simulink model "risingEdge"  (R2024a)
settings: Solver=FixedStepDiscrete  StartTime=0.0  StopTime=10.0  RelTol=1e-3
undefined symbols (not defined in the file): HDL_ieee_8021513, rising_edge_detector
settings Model: DataTypeOverride=Off  Creator=cotti  LastModifiedBy=cotti
settings OptimizationCC: BlockReduction=off  ConditionallyExecuteInputs=off  DefaultParameterBehavior=Inlined  InheritOutputTypeSmallerThanSingle=on
settings DebuggingCC: AlgebraicLoopMsg=error  ArtificialAlgebraicLoopMsg=error  SingleTaskRateTransMsg=error  UnconnectedInputMsg=warning  UnconnectedOutputMsg=warning  UnconnectedLineMsg=warning
settings HardwareCC: ProdBitPerPointer=32  ProdBitPerSizeT=32  ProdBitPerPtrDiffT=32  ProdLargestAtomicFloat=None  ProdIntDivRoundTo=Undefined  ProdEndianess=Unspecified  ProdWordSize=32  ProdHWDeviceType=ASIC/FPGA->ASIC/FPGA  TargetBitPerLong=64  TargetBitPerPointer=64  TargetBitPerSizeT=64  TargetBitPerPtrDiffT=64  TargetLongLongMode=on  TargetIntDivRoundTo=Zero  TargetEndianess=LittleEndian  TargetWordSize=64  TargetHWDeviceType=Custom Processor->MATLAB Host Computer  ProdEqTarget=off

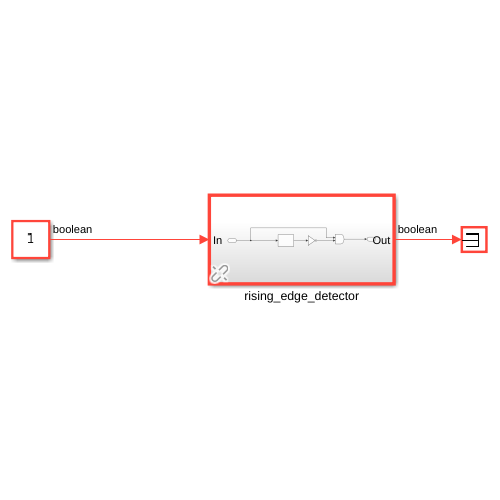
[thumbnail: Simulink's stored preview of the top-level diagram]
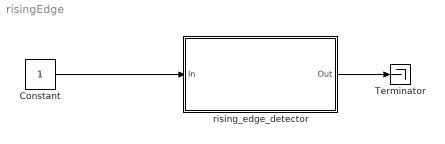
== system risingEdge ==
  Constant : Constant  OutDataTypeStr=boolean  SampleTime=1
  Terminator : Terminator
  rising_edge_detector : Subsystem  AncestorBlock=HDL_ieee_8021513/rising_edge_detector  TreatAsAtomicUnit=on
  wires:
  rising_edge_detector/1(Out) -> Terminator/1
  Constant/1 -> rising_edge_detector/1(In)

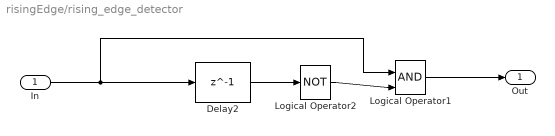
== system risingEdge/rising_edge_detector ==
  In : Inport
  Delay2 : Delay  DelayLength=1  InitialCondition=0  UseCircularBuffer=on
  Logical Operator1 : Logic  IconShape=distinctive  AllPortsSameDT=off  OutDataTypeStr=boolean
  Logical Operator2 : Logic  Operator=NOT  IconShape=distinctive  AllPortsSameDT=off  OutDataTypeStr=boolean
  Out : Outport
  wires:
  Logical Operator1/1 -> Out/1
  In/1 -> Delay2/1, Logical Operator1/1
  Delay2/1 -> Logical Operator2/1
  Logical Operator2/1 -> Logical Operator1/2
